simulink model "angle_to_pwm"  (R2017a)
settings: Solver=VariableStepAuto  StartTime=0.0  StopTime=3000  RelTol=1e-3
libraries: hdlsllib x2
settings Model: Creator=Ryan Corkery  LastModifiedBy=Ryan Corkery

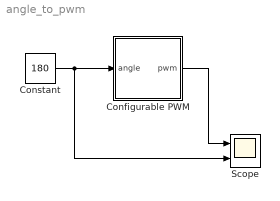
== system angle_to_pwm ==
  Configurable PWM : Subsystem
  Constant : Constant  Value=180  OutDataTypeStr=uint8
  Scope : Scope  NumInputPorts=2
  wires:
  Configurable PWM/1(pwm) -> Scope/1
  Constant/1 -> Scope/2, Configurable PWM/1("angle ")

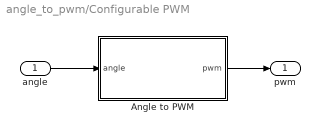
== system angle_to_pwm/Configurable PWM ==
  "angle " : Inport  OutDataTypeStr=uint8
  Angle to PWM : Subsystem
  pwm : Outport
  wires:
  "angle "/1 -> Angle to PWM/1("angle ")
  Angle to PWM/1(pwm) -> pwm/1

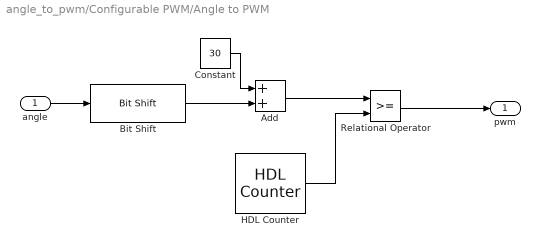
== system angle_to_pwm/Configurable PWM/Angle to PWM ==
  "angle " : Inport  OutDataTypeStr=uint8
  Add : Sum
  Bit Shift : hdlsllib/HDL Operations/Bit Shift  mode=Shift Right Logical  N=1
      settings: SourceProductName=HDL Coder  SourceProductBaseCode=HD
  Constant : Constant  Value=30  OutDataTypeStr=uint8
  HDL Counter : hdlsllib/HDL Operations/HDL Counter  CountType=Count limited  CountInit=0  CountStep=1  CountMax=1000  CountFromType=Initial value  CountFrom=0  CountResetPort=off  CountLoadPort=off  CountEnbPort=off  CountDirPort=off  CountDataType=Unsigned  CountWordLen=16  CountFracLen=0  CountSampTime=1
      settings: SourceProductName=HDL Coder  SourceProductBaseCode=HD
  Relational Operator : RelationalOperator  OutDataTypeStr=boolean  RndMeth=Simplest
  pwm : Outport
  wires:
  HDL Counter/1 -> Relational Operator/2
  Relational Operator/1 -> pwm/1
  Add/1 -> Relational Operator/1
  Bit Shift/1 -> Add/2
  Constant/1 -> Add/1
  "angle "/1 -> Bit Shift/1
